simulink model "modellab1"  (R2023a)
settings: Solver=VariableStepAuto  StartTime=0.0  StopTime=0.25  RelTol=1e-3
values from neighbouring files (symbols this model uses):
  B = 0.001    [scrlab1.m]
  Cm = 1.3    [scrlab1.m]
  Cv = 3.15    [scrlab1.m]
  J = 7*(10^(-6))    (= 7e-06)    [scrlab1.m]
  La = 0.0015    [scrlab1.m]
  Lo = 0.013    [scrlab1.m]
  Ra = 8    [scrlab1.m]
settings Model: Creator=desire  LastModifiedBy=desire

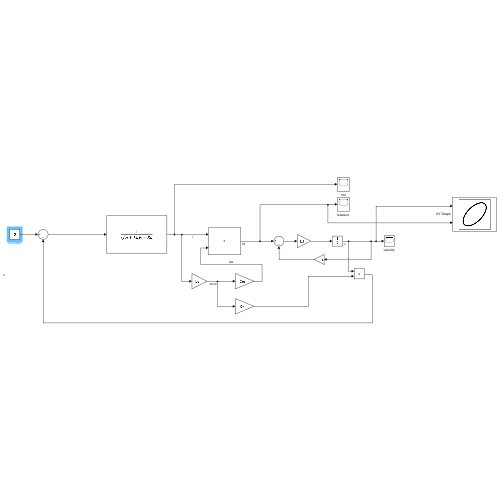
[thumbnail: Simulink's stored preview of the top-level diagram]
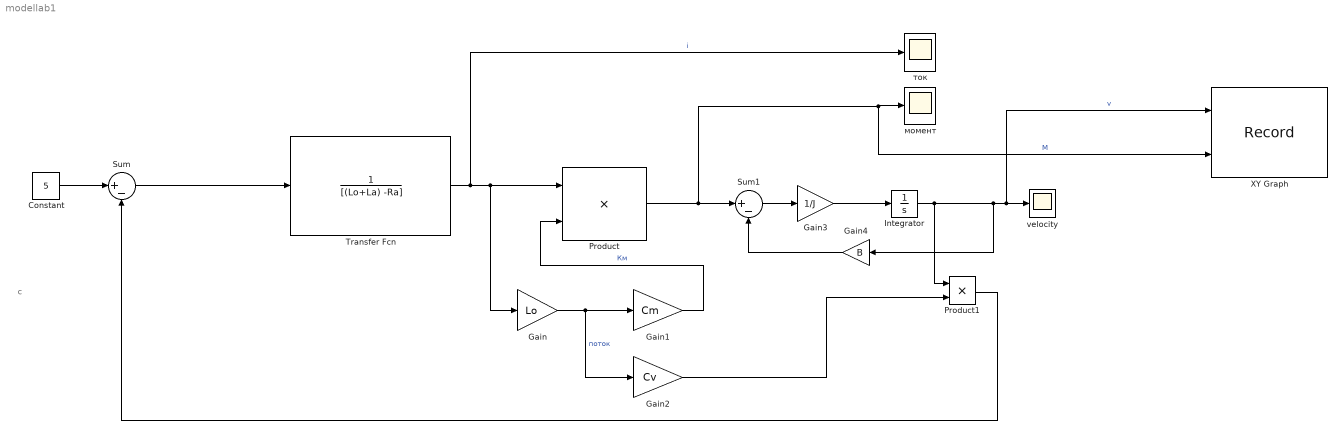
== system modellab1 ==
  note: c
  Constant : Constant  Value=5
  Gain : Gain  Gain=Lo
  Gain1 : Gain  Gain=Cm
  Gain2 : Gain  Gain=Cv
  Gain3 : Gain  Gain=1/J
  Gain4 : Gain  Gain=B
  Integrator : Integrator
  Product : Product
  Product1 : Product
  Sum : Sum  Inputs=|+-
  Sum1 : Sum  Inputs=|+-
  Transfer Fcn : TransferFcn  Denominator=[(Lo+La) -Ra]
  XY Graph : Record  FileSettingsInternal="{\"entries\":[{\"content\":{\"excelSettings\":{\"content\":{},\"type\":\"Streamout.ExcelSettings\"}},\"type\":\"Streamout.FileSettingStorage\",\"uuid\":\"e678f825-0787-4e8e-ac47-7cb9cacd380b\"}],\"packageUris\":[\"http://schema.mathworks.com/mf0/streamout_blocks/R2020a\"],\"version\":\"1.0\"}"  Layout=[1 1]  SignalsInternal="{\"entries\":[{\"content\":{\"signals\":[{\"content\":{\"blockPath\":[\"modellab1/XY Graph\"],\"dimensions\":[1],\"domain\":\"modellab1/XY Graph\",\"lineColor\":\"#a2142f\",\"plots\":[1],\"port\":1,\"sid\":[\"\"],\"signalID\":203,\"signalName\":\"v\"},\"type\":\"RecordBlkView.Signal\",\"uuid\":\"22faf2ff-8fc6-4ba1-8388-530d5a3a2f96\"},{\"content\":{\"blockPath\":[\"modellab1/XY Graph\"],\"dimensions\":[1],\"domain\":\"modellab1/XY Graph\",\"lineColor\":\"#139fff\",\"plots\":[1],\"port\":2,\"sid\":[\"\"],\"signalID\":207,\"signalName\":\"M\"},\"type\":\"RecordBlkView.Signal\",\"uuid\":\"160c9586-95f5-4c11-b6c1-6e8c1b47a80c\"}]},\"type\":\"RecordBlkView.InputSignals\",\"uuid\":\"3776b16f-9f99-4afd-8726-80263f7dd2c3\"}],\"packageUris\":[\"http://schema.mathworks.com/mf0/streamout_blocks/R2020a\"],\"version\":\"1.0\"}"  VisualizationBindings="{\"xyplotplugin\":{\"info\":[{\"series\":[{\"bindingParametersList\":[{\"parameter\":\"X-Axis\",\"signalID\":203,\"signalName\":\"v\"},{\"parameter\":\"Y-Axis\",\"signalID\":207,\"signalName\":\"M\"}],\"seriesID\":54620}],\"subplotID\":1}]}}"  CompatibilityTag=XY
  velocity : Scope
  момент : Scope
  ток : Scope
  wires:
  Constant/1 -> Sum/1
  Sum/1 -> Transfer Fcn/1
  Transfer Fcn/1 -> ток/1, Gain/1, Product/1  "i"
  Gain/1 -> Gain2/1, Gain1/1  "поток"
  Gain1/1 -> Product/2  "Км"
  Product/1 -> XY Graph/2, момент/1, Sum1/1  "M"
  Sum1/1 -> Gain3/1
  Gain3/1 -> Integrator/1
  Integrator/1 -> Gain4/1, XY Graph/1, velocity/1, Product1/1  "v"
  Gain2/1 -> Product1/2
  Product1/1 -> Sum/2
  Gain4/1 -> Sum1/2
